simulink model "suspension"  (R2024a)
settings: Solver=VariableStepAuto  StartTime=0.0  StopTime=90.0  RelTol=1e-3
InitFcn:
  | parseLogs
model workspace (MAT data in the model file):
  valve_open = 0.5
libraries: cstblocks x1
settings Model: Creator=volubepossum  LastModifiedBy=mikom

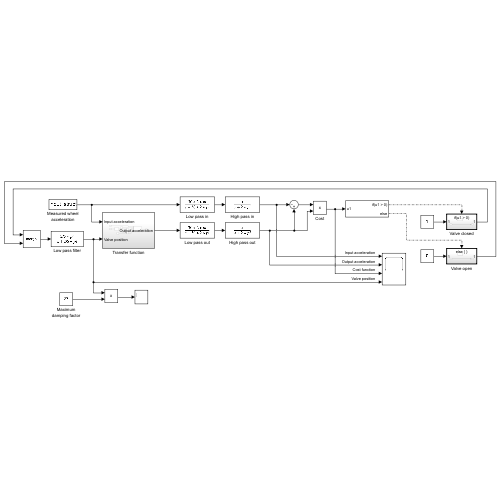
[thumbnail: Simulink's stored preview of the top-level diagram]
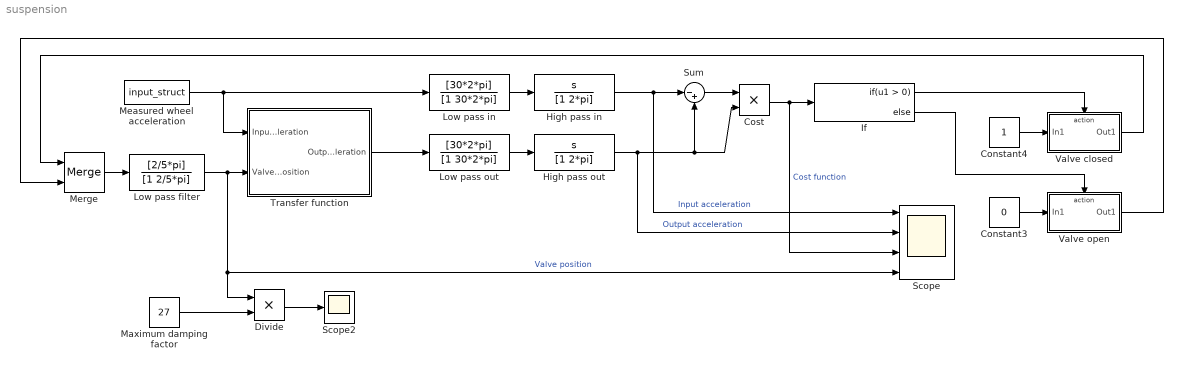
== system suspension ==
  Constant3 : Constant  Value=0
  Constant4 : Constant
  Cost : Product  Inputs=**
  Divide : Product  Inputs=**
  High pass in : TransferFcn  Numerator=[1 0]  Denominator=[1 2*pi]
  High pass out : TransferFcn  Numerator=[1 0]  Denominator=[1 2*pi]
  If : If
  Low pass filter : TransferFcn  Numerator=[2/5*pi]  Denominator=[1 2/5*pi]
  Low pass in : TransferFcn  Numerator=[30*2*pi]  Denominator=[1 30*2*pi]
  Low pass out : TransferFcn  Numerator=[30*2*pi]  Denominator=[1 30*2*pi]
  Maximum damping factor : Constant  Value=27
  Measured wheel acceleration : FromWorkspace  VariableName=input_struct
  Merge : Merge
  Scope : Scope  NumInputPorts=4
  Scope2 : Scope
  Sum : Sum  Inputs=|-+
  Transfer function : Subsystem
  Valve closed : Subsystem  TreatAsAtomicUnit=on
  Valve open : Subsystem  TreatAsAtomicUnit=on
  wires:
  Low pass out/1 -> High pass out/1
  Transfer function/1(Output acceleration) -> Low pass out/1
  Measured wheel acceleration/1 -> Low pass in/1, Transfer function/1(Input acceleration)
  Low pass in/1 -> High pass in/1
  High pass out/1 -> Sum/2, Cost/2, Scope/2  "Output acceleration"
  High pass in/1 -> Scope/1, Sum/1  "Input acceleration"
  Sum/1 -> Cost/1
  Cost/1 -> Scope/3, If/1  "Cost function"
  Valve open/1(Out1) -> Merge/2
  Valve closed/1(Out1) -> Merge/1
  Merge/1 -> Low pass filter/1
  If/2 -> Valve open/Action
  Constant3/1 -> Valve open/1(In1)
  If/1 -> Valve closed/Action
  Constant4/1 -> Valve closed/1(In1)
  Low pass filter/1 -> Scope/4, Divide/1, Transfer function/2(Valve position)  "Valve position"
  Maximum damping factor/1 -> Divide/2
  Divide/1 -> Scope2/1

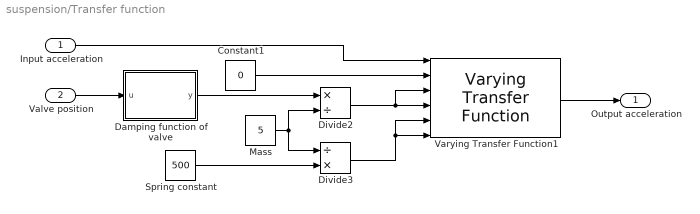
== system suspension/Transfer function ==
  Input acceleration : Inport
  Valve position : Inport  Port=2
  Constant1 : Constant  Value=0
  Damping function of valve : MATLAB Function  TreatAsAtomicUnit=on
  Divide2 : Product  Inputs=*/
  Divide3 : Product  Inputs=/*
  Mass : Constant  Value=5
  Spring constant : Constant  Value=500
  Varying Transfer Function1 : cstblocks/Linear Parameter Varying/Varying Transfer Function  N=2  Feedthrough=on
  Output acceleration : Outport
  wires:
  Divide3/1 -> Varying Transfer Function1/5, Varying Transfer Function1/6
  Spring constant/1 -> Divide3/2
  Constant1/1 -> Varying Transfer Function1/2
  Input acceleration/1 -> Varying Transfer Function1/1
  Divide2/1 -> Varying Transfer Function1/4, Varying Transfer Function1/3
  Damping function of valve/1(y) -> Divide2/1
  Varying Transfer Function1/1 -> Output acceleration/1
  Valve position/1 -> Damping function of valve/1(u)
  Mass/1 -> Divide3/1, Divide2/2

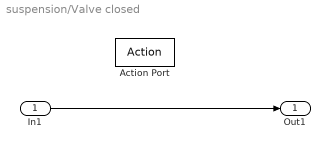
== system suspension/Valve closed ==
  In1 : Inport
  Action Port : ActionPort  ActionPortLabel=if(u1 > 0)
  Out1 : Outport
  wires:
  In1/1 -> Out1/1

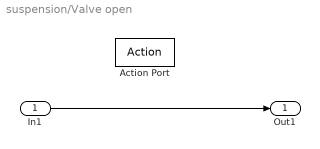
== system suspension/Valve open ==
  In1 : Inport
  Action Port : ActionPort  ActionPortLabel=else
  Out1 : Outport
  wires:
  In1/1 -> Out1/1

== matlab function suspension/Transfer function/Damping function of valve ==
  data: u input; y output
function y = fcn(u)
y = 27*u;
